simulink model "Task3"  (R2025a)
settings: Solver=VariableStepAuto  StartTime=0.0  StopTime=5  RelTol=1e-3
undefined symbols (not defined in the file or in its folder): Kc
settings Model: Creator=sunzi  LastModifiedBy=sunzi

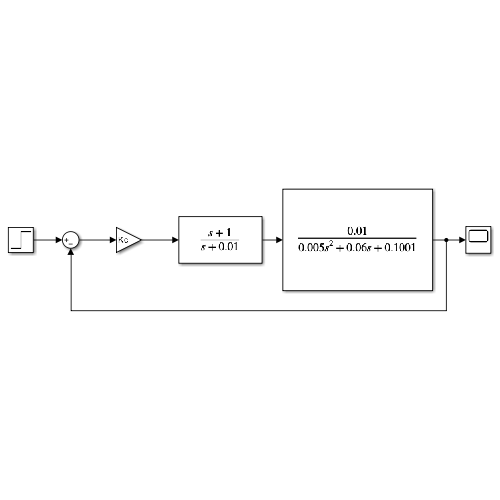
[thumbnail: Simulink's stored preview of the top-level diagram]
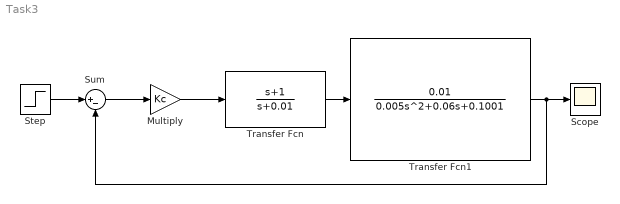
== system Task3 ==
  Multiply : Gain  Gain=Kc
  Scope : Scope
      settings: ActiveDisplayYMinimum=-0.14293759714620477  ActiveDisplayYMaximum=1.2864383743158432
  Step : Step  Time=0  SampleTime=0
  Sum : Sum  Inputs=|+-
  Transfer Fcn : TransferFcn  Numerator=[1 1]  Denominator=[1 0.01]
  Transfer Fcn1 : TransferFcn  Numerator=[0.01]  Denominator=[0.005 0.06 0.1001]
  wires:
  Multiply/1 -> Transfer Fcn/1
  Transfer Fcn/1 -> Transfer Fcn1/1
  Sum/1 -> Multiply/1
  Step/1 -> Sum/1
  Transfer Fcn1/1 -> Sum/2, Scope/1
